simulink model "erro"  (R2022a)
settings: Solver=VariableStepAuto  StartTime=0.0  StopTime=10.0  RelTol=1e-3
libraries: simulink x1
settings Model: Creator=a2150336  LastModifiedBy=a2150336

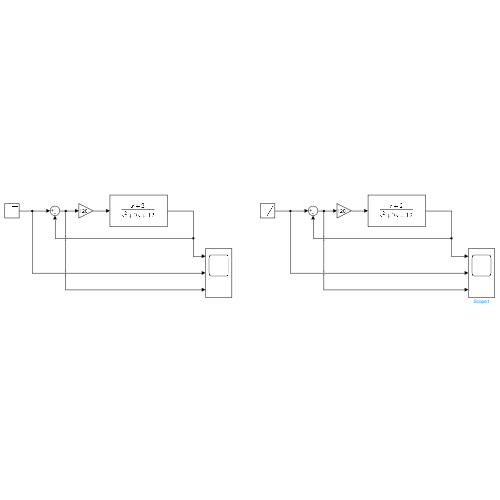
[thumbnail: Simulink's stored preview of the top-level diagram]
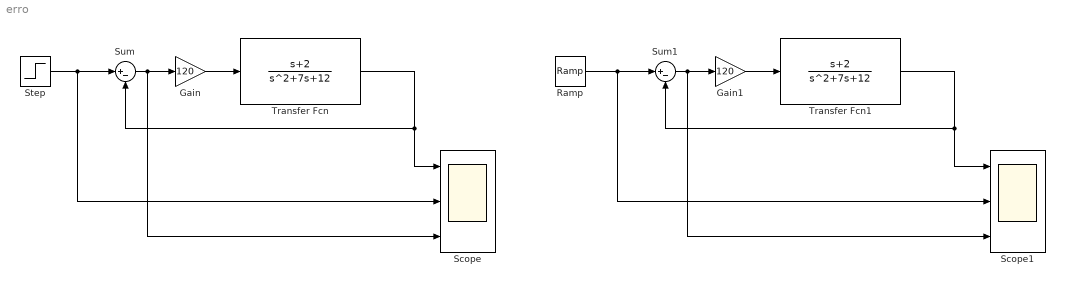
== system erro ==
  Gain : Gain  Gain=120
  Gain1 : Gain  Gain=120
  Ramp : simulink/Sources/Ramp  slope=5  start=0  InitialOutput=0
  Scope : Scope  NumInputPorts=3
  Scope1 : Scope  NumInputPorts=3
  Step : Step  After=5  SampleTime=0
  Sum : Sum  Inputs=|+-
  Sum1 : Sum  Inputs=|+-
  Transfer Fcn : TransferFcn  Numerator=[1 2]  Denominator=[1 7 12]
  Transfer Fcn1 : TransferFcn  Numerator=[1 2]  Denominator=[1 7 12]
  wires:
  Gain/1 -> Transfer Fcn/1
  Transfer Fcn/1 -> Sum/2, Scope/1
  Sum/1 -> Scope/3, Gain/1
  Step/1 -> Scope/2, Sum/1
  Transfer Fcn1/1 -> Sum1/2, Scope1/1
  Ramp/1 -> Scope1/2, Sum1/1
  Sum1/1 -> Scope1/3, Gain1/1
  Gain1/1 -> Transfer Fcn1/1
